simulink model "gm_rec_i2s"  (R2023b)
settings: Solver=VariableStepAuto  StartTime=0.0  StopTime=20  RelTol=1e-3
undefined symbols (not defined in the file or in its folder): cnt1_LRCLK, cnt2_SCLK
libraries: hdlsllib x4
(part 3 of 4)

== system gm_rec_i2s/REC_I2S_NOFIFO/Subsystem1/SIPO_16BIT/SIPO_8BIT/SIPO_4BIT/SIPO_2BIT ==
  SERIAL_IN : Inport  OutDataTypeStr=boolean
  ENABLE : Inport  Port=2
  Bus Creator : BusCreator  Inputs=2
  Delay : Delay  DelayLength=1  InitialCondition=0  ShowEnablePort=on
      settings: InputPortMap=u0,e6
  Delay1 : Delay  DelayLength=1  InitialCondition=0  ShowEnablePort=on
      settings: InputPortMap=u0,e6
  PARA_OUT : Outport  OutDataTypeStr=boolean  VectorParamsAs1DForOutWhenUnconnected=off
  SERIAL_OUT : Outport  Port=2  OutDataTypeStr=boolean  VectorParamsAs1DForOutWhenUnconnected=off
  wires:
  Bus Creator/1 -> PARA_OUT/1
  Delay/1 -> Delay1/1, Bus Creator/2
  Delay1/1 -> Bus Creator/1, SERIAL_OUT/1
  ENABLE/1 -> Delay/2, Delay1/2
  SERIAL_IN/1 -> Delay/1

== system gm_rec_i2s/REC_I2S_NOFIFO/Subsystem1/SIPO_16BIT/SIPO_8BIT/SIPO_4BIT/SIPO_2BIT1 ==
  SERIAL_IN : Inport
  ENABLE : Inport  Port=2
  Bus Creator : BusCreator  Inputs=2
  Delay : Delay  DelayLength=1  InitialCondition=0  ShowEnablePort=on
      settings: InputPortMap=u0,e6
  Delay1 : Delay  DelayLength=1  InitialCondition=0  ShowEnablePort=on
      settings: InputPortMap=u0,e6
  PARA_OUT : Outport  VectorParamsAs1DForOutWhenUnconnected=off
  SERIAL_OUT : Outport  Port=2  VectorParamsAs1DForOutWhenUnconnected=off
  wires:
  Bus Creator/1 -> PARA_OUT/1
  Delay/1 -> Delay1/1, Bus Creator/2
  Delay1/1 -> Bus Creator/1, SERIAL_OUT/1
  ENABLE/1 -> Delay/2, Delay1/2
  SERIAL_IN/1 -> Delay/1

== system gm_rec_i2s/REC_I2S_NOFIFO/Subsystem1/SIPO_16BIT/SIPO_8BIT/SIPO_4BIT1/SIPO_2BIT ==
  SERIAL_IN : Inport
  ENABLE : Inport  Port=2
  Bus Creator : BusCreator  Inputs=2
  Delay : Delay  DelayLength=1  InitialCondition=0  ShowEnablePort=on
      settings: InputPortMap=u0,e6
  Delay1 : Delay  DelayLength=1  InitialCondition=0  ShowEnablePort=on
      settings: InputPortMap=u0,e6
  PARA_OUT : Outport  VectorParamsAs1DForOutWhenUnconnected=off
  SERIAL_OUT : Outport  Port=2  VectorParamsAs1DForOutWhenUnconnected=off
  wires:
  Bus Creator/1 -> PARA_OUT/1
  Delay/1 -> Delay1/1, Bus Creator/2
  Delay1/1 -> Bus Creator/1, SERIAL_OUT/1
  ENABLE/1 -> Delay/2, Delay1/2
  SERIAL_IN/1 -> Delay/1

== system gm_rec_i2s/REC_I2S_NOFIFO/Subsystem1/SIPO_16BIT/SIPO_8BIT/SIPO_4BIT1/SIPO_2BIT1 ==
  SERIAL_IN : Inport
  ENABLE : Inport  Port=2
  Bus Creator : BusCreator  Inputs=2
  Delay : Delay  DelayLength=1  InitialCondition=0  ShowEnablePort=on
      settings: InputPortMap=u0,e6
  Delay1 : Delay  DelayLength=1  InitialCondition=0  ShowEnablePort=on
      settings: InputPortMap=u0,e6
  PARA_OUT : Outport  VectorParamsAs1DForOutWhenUnconnected=off
  SERIAL_OUT : Outport  Port=2  VectorParamsAs1DForOutWhenUnconnected=off
  wires:
  Bus Creator/1 -> PARA_OUT/1
  Delay/1 -> Delay1/1, Bus Creator/2
  Delay1/1 -> Bus Creator/1, SERIAL_OUT/1
  ENABLE/1 -> Delay/2, Delay1/2
  SERIAL_IN/1 -> Delay/1

== system gm_rec_i2s/REC_I2S_NOFIFO/Subsystem1/SIPO_16BIT/SIPO_8BIT1/SIPO_4BIT/SIPO_2BIT ==
  SERIAL_IN : Inport
  ENABLE : Inport  Port=2
  Bus Creator : BusCreator  Inputs=2
  Delay : Delay  DelayLength=1  InitialCondition=0  ShowEnablePort=on
      settings: InputPortMap=u0,e6
  Delay1 : Delay  DelayLength=1  InitialCondition=0  ShowEnablePort=on
      settings: InputPortMap=u0,e6
  PARA_OUT : Outport  VectorParamsAs1DForOutWhenUnconnected=off
  SERIAL_OUT : Outport  Port=2  VectorParamsAs1DForOutWhenUnconnected=off
  wires:
  Bus Creator/1 -> PARA_OUT/1
  Delay/1 -> Delay1/1, Bus Creator/2
  Delay1/1 -> Bus Creator/1, SERIAL_OUT/1
  ENABLE/1 -> Delay/2, Delay1/2
  SERIAL_IN/1 -> Delay/1

== system gm_rec_i2s/REC_I2S_NOFIFO/Subsystem1/SIPO_16BIT/SIPO_8BIT1/SIPO_4BIT/SIPO_2BIT1 ==
  SERIAL_IN : Inport
  ENABLE : Inport  Port=2
  Bus Creator : BusCreator  Inputs=2
  Delay : Delay  DelayLength=1  InitialCondition=0  ShowEnablePort=on
      settings: InputPortMap=u0,e6
  Delay1 : Delay  DelayLength=1  InitialCondition=0  ShowEnablePort=on
      settings: InputPortMap=u0,e6
  PARA_OUT : Outport  VectorParamsAs1DForOutWhenUnconnected=off
  SERIAL_OUT : Outport  Port=2  VectorParamsAs1DForOutWhenUnconnected=off
  wires:
  Bus Creator/1 -> PARA_OUT/1
  Delay/1 -> Delay1/1, Bus Creator/2
  Delay1/1 -> Bus Creator/1, SERIAL_OUT/1
  ENABLE/1 -> Delay/2, Delay1/2
  SERIAL_IN/1 -> Delay/1

== system gm_rec_i2s/REC_I2S_NOFIFO/Subsystem1/SIPO_16BIT/SIPO_8BIT1/SIPO_4BIT1/SIPO_2BIT ==
  SERIAL_IN : Inport
  ENABLE : Inport  Port=2
  Bus Creator : BusCreator  Inputs=2
  Delay : Delay  DelayLength=1  InitialCondition=0  ShowEnablePort=on
      settings: InputPortMap=u0,e6
  Delay1 : Delay  DelayLength=1  InitialCondition=0  ShowEnablePort=on
      settings: InputPortMap=u0,e6
  PARA_OUT : Outport  VectorParamsAs1DForOutWhenUnconnected=off
  SERIAL_OUT : Outport  Port=2  VectorParamsAs1DForOutWhenUnconnected=off
  wires:
  Bus Creator/1 -> PARA_OUT/1
  Delay/1 -> Delay1/1, Bus Creator/2
  Delay1/1 -> Bus Creator/1, SERIAL_OUT/1
  ENABLE/1 -> Delay/2, Delay1/2
  SERIAL_IN/1 -> Delay/1

== system gm_rec_i2s/REC_I2S_NOFIFO/Subsystem1/SIPO_16BIT/SIPO_8BIT1/SIPO_4BIT1/SIPO_2BIT1 ==
  SERIAL_IN : Inport
  ENABLE : Inport  Port=2
  Bus Creator : BusCreator  Inputs=2
  Delay : Delay  DelayLength=1  InitialCondition=0  ShowEnablePort=on
      settings: InputPortMap=u0,e6
  Delay1 : Delay  DelayLength=1  InitialCondition=0  ShowEnablePort=on
      settings: InputPortMap=u0,e6
  PARA_OUT : Outport  VectorParamsAs1DForOutWhenUnconnected=off
  SERIAL_OUT : Outport  Port=2  VectorParamsAs1DForOutWhenUnconnected=off
  wires:
  Bus Creator/1 -> PARA_OUT/1
  Delay/1 -> Delay1/1, Bus Creator/2
  Delay1/1 -> Bus Creator/1, SERIAL_OUT/1
  ENABLE/1 -> Delay/2, Delay1/2
  SERIAL_IN/1 -> Delay/1

== system gm_rec_i2s/REC_I2S_NOFIFO/Subsystem1/SIPO_16BIT1/SIPO_8BIT/SIPO_4BIT/SIPO_2BIT ==
  SERIAL_IN : Inport  OutDataTypeStr=boolean
  ENABLE : Inport  Port=2
  Bus Creator : BusCreator  Inputs=2
  Delay : Delay  DelayLength=1  InitialCondition=0  ShowEnablePort=on
      settings: InputPortMap=u0,e6
  Delay1 : Delay  DelayLength=1  InitialCondition=0  ShowEnablePort=on
      settings: InputPortMap=u0,e6
  PARA_OUT : Outport  OutDataTypeStr=boolean  VectorParamsAs1DForOutWhenUnconnected=off
  SERIAL_OUT : Outport  Port=2  OutDataTypeStr=boolean  VectorParamsAs1DForOutWhenUnconnected=off
  wires:
  Bus Creator/1 -> PARA_OUT/1
  Delay/1 -> Delay1/1, Bus Creator/2
  Delay1/1 -> Bus Creator/1, SERIAL_OUT/1
  ENABLE/1 -> Delay/2, Delay1/2
  SERIAL_IN/1 -> Delay/1

== system gm_rec_i2s/REC_I2S_NOFIFO/Subsystem1/SIPO_16BIT1/SIPO_8BIT/SIPO_4BIT/SIPO_2BIT1 ==
  SERIAL_IN : Inport
  ENABLE : Inport  Port=2
  Bus Creator : BusCreator  Inputs=2
  Delay : Delay  DelayLength=1  InitialCondition=0  ShowEnablePort=on
      settings: InputPortMap=u0,e6
  Delay1 : Delay  DelayLength=1  InitialCondition=0  ShowEnablePort=on
      settings: InputPortMap=u0,e6
  PARA_OUT : Outport  VectorParamsAs1DForOutWhenUnconnected=off
  SERIAL_OUT : Outport  Port=2  VectorParamsAs1DForOutWhenUnconnected=off
  wires:
  Bus Creator/1 -> PARA_OUT/1
  Delay/1 -> Delay1/1, Bus Creator/2
  Delay1/1 -> Bus Creator/1, SERIAL_OUT/1
  ENABLE/1 -> Delay/2, Delay1/2
  SERIAL_IN/1 -> Delay/1

== system gm_rec_i2s/REC_I2S_NOFIFO/Subsystem1/SIPO_16BIT1/SIPO_8BIT/SIPO_4BIT1/SIPO_2BIT ==
  SERIAL_IN : Inport
  ENABLE : Inport  Port=2
  Bus Creator : BusCreator  Inputs=2
  Delay : Delay  DelayLength=1  InitialCondition=0  ShowEnablePort=on
      settings: InputPortMap=u0,e6
  Delay1 : Delay  DelayLength=1  InitialCondition=0  ShowEnablePort=on
      settings: InputPortMap=u0,e6
  PARA_OUT : Outport  VectorParamsAs1DForOutWhenUnconnected=off
  SERIAL_OUT : Outport  Port=2  VectorParamsAs1DForOutWhenUnconnected=off
  wires:
  Bus Creator/1 -> PARA_OUT/1
  Delay/1 -> Delay1/1, Bus Creator/2
  Delay1/1 -> Bus Creator/1, SERIAL_OUT/1
  ENABLE/1 -> Delay/2, Delay1/2
  SERIAL_IN/1 -> Delay/1

== system gm_rec_i2s/REC_I2S_NOFIFO/Subsystem1/SIPO_16BIT1/SIPO_8BIT/SIPO_4BIT1/SIPO_2BIT1 ==
  SERIAL_IN : Inport
  ENABLE : Inport  Port=2
  Bus Creator : BusCreator  Inputs=2
  Delay : Delay  DelayLength=1  InitialCondition=0  ShowEnablePort=on
      settings: InputPortMap=u0,e6
  Delay1 : Delay  DelayLength=1  InitialCondition=0  ShowEnablePort=on
      settings: InputPortMap=u0,e6
  PARA_OUT : Outport  VectorParamsAs1DForOutWhenUnconnected=off
  SERIAL_OUT : Outport  Port=2  VectorParamsAs1DForOutWhenUnconnected=off
  wires:
  Bus Creator/1 -> PARA_OUT/1
  Delay/1 -> Delay1/1, Bus Creator/2
  Delay1/1 -> Bus Creator/1, SERIAL_OUT/1
  ENABLE/1 -> Delay/2, Delay1/2
  SERIAL_IN/1 -> Delay/1

== system gm_rec_i2s/REC_I2S_NOFIFO/Subsystem1/SIPO_16BIT1/SIPO_8BIT1/SIPO_4BIT/SIPO_2BIT ==
  SERIAL_IN : Inport
  ENABLE : Inport  Port=2
  Bus Creator : BusCreator  Inputs=2
  Delay : Delay  DelayLength=1  InitialCondition=0  ShowEnablePort=on
      settings: InputPortMap=u0,e6
  Delay1 : Delay  DelayLength=1  InitialCondition=0  ShowEnablePort=on
      settings: InputPortMap=u0,e6
  PARA_OUT : Outport  VectorParamsAs1DForOutWhenUnconnected=off
  SERIAL_OUT : Outport  Port=2  VectorParamsAs1DForOutWhenUnconnected=off
  wires:
  Bus Creator/1 -> PARA_OUT/1
  Delay/1 -> Delay1/1, Bus Creator/2
  Delay1/1 -> Bus Creator/1, SERIAL_OUT/1
  ENABLE/1 -> Delay/2, Delay1/2
  SERIAL_IN/1 -> Delay/1

== system gm_rec_i2s/REC_I2S_NOFIFO/Subsystem1/SIPO_16BIT1/SIPO_8BIT1/SIPO_4BIT/SIPO_2BIT1 ==
  SERIAL_IN : Inport
  ENABLE : Inport  Port=2
  Bus Creator : BusCreator  Inputs=2
  Delay : Delay  DelayLength=1  InitialCondition=0  ShowEnablePort=on
      settings: InputPortMap=u0,e6
  Delay1 : Delay  DelayLength=1  InitialCondition=0  ShowEnablePort=on
      settings: InputPortMap=u0,e6
  PARA_OUT : Outport  VectorParamsAs1DForOutWhenUnconnected=off
  SERIAL_OUT : Outport  Port=2  VectorParamsAs1DForOutWhenUnconnected=off
  wires:
  Bus Creator/1 -> PARA_OUT/1
  Delay/1 -> Delay1/1, Bus Creator/2
  Delay1/1 -> Bus Creator/1, SERIAL_OUT/1
  ENABLE/1 -> Delay/2, Delay1/2
  SERIAL_IN/1 -> Delay/1

== system gm_rec_i2s/REC_I2S_NOFIFO/Subsystem1/SIPO_16BIT1/SIPO_8BIT1/SIPO_4BIT1/SIPO_2BIT ==
  SERIAL_IN : Inport
  ENABLE : Inport  Port=2
  Bus Creator : BusCreator  Inputs=2
  Delay : Delay  DelayLength=1  InitialCondition=0  ShowEnablePort=on
      settings: InputPortMap=u0,e6
  Delay1 : Delay  DelayLength=1  InitialCondition=0  ShowEnablePort=on
      settings: InputPortMap=u0,e6
  PARA_OUT : Outport  VectorParamsAs1DForOutWhenUnconnected=off
  SERIAL_OUT : Outport  Port=2  VectorParamsAs1DForOutWhenUnconnected=off
  wires:
  Bus Creator/1 -> PARA_OUT/1
  Delay/1 -> Delay1/1, Bus Creator/2
  Delay1/1 -> Bus Creator/1, SERIAL_OUT/1
  ENABLE/1 -> Delay/2, Delay1/2
  SERIAL_IN/1 -> Delay/1

== system gm_rec_i2s/REC_I2S_NOFIFO/Subsystem1/SIPO_16BIT1/SIPO_8BIT1/SIPO_4BIT1/SIPO_2BIT1 ==
  SERIAL_IN : Inport
  ENABLE : Inport  Port=2
  Bus Creator : BusCreator  Inputs=2
  Delay : Delay  DelayLength=1  InitialCondition=0  ShowEnablePort=on
      settings: InputPortMap=u0,e6
  Delay1 : Delay  DelayLength=1  InitialCondition=0  ShowEnablePort=on
      settings: InputPortMap=u0,e6
  PARA_OUT : Outport  VectorParamsAs1DForOutWhenUnconnected=off
  SERIAL_OUT : Outport  Port=2  VectorParamsAs1DForOutWhenUnconnected=off
  wires:
  Bus Creator/1 -> PARA_OUT/1
  Delay/1 -> Delay1/1, Bus Creator/2
  Delay1/1 -> Bus Creator/1, SERIAL_OUT/1
  ENABLE/1 -> Delay/2, Delay1/2
  SERIAL_IN/1 -> Delay/1

== system gm_rec_i2s/REC_I2S_FIFO/SIPO_32BIT_L/Subsystem/SIPO_16BIT/SIPO_8BIT/SIPO_4BIT/2BIT_SIPO ==
  SERIAL_IN : Inport
  Constant : Constant  OutDataTypeStr=boolean  SampleTime=-1
  Delay : Delay  DelayLength=1  InitialCondition=0  ShowEnablePort=on
      settings: InputPortMap=u0,e6
  Delay1 : Delay  DelayLength=1  InitialCondition=0  ShowEnablePort=on
      settings: InputPortMap=u0,e6
  Vector Concatenate : Concatenate
  PARA_OUT : Outport  VectorParamsAs1DForOutWhenUnconnected=off
  SERIAL_OUT : Outport  Port=2  VectorParamsAs1DForOutWhenUnconnected=off
  wires:
  SERIAL_IN/1 -> Delay/1
  Delay1/1 -> SERIAL_OUT/1, Vector Concatenate/1
  Vector Concatenate/1 -> PARA_OUT/1
  Delay/1 -> Vector Concatenate/2, Delay1/1
  Constant/1 -> Delay1/2, Delay/2

== system gm_rec_i2s/REC_I2S_FIFO/SIPO_32BIT_L/Subsystem/SIPO_16BIT/SIPO_8BIT/SIPO_4BIT/2BIT_SIPO1 ==
  SERIAL_IN : Inport
  Constant : Constant  OutDataTypeStr=boolean  SampleTime=-1
  Delay : Delay  DelayLength=1  InitialCondition=0  ShowEnablePort=on
      settings: InputPortMap=u0,e6
  Delay1 : Delay  DelayLength=1  InitialCondition=0  ShowEnablePort=on
      settings: InputPortMap=u0,e6
  Vector Concatenate : Concatenate
  PARA_OUT : Outport  VectorParamsAs1DForOutWhenUnconnected=off
  SERIAL_OUT : Outport  Port=2  VectorParamsAs1DForOutWhenUnconnected=off
  wires:
  SERIAL_IN/1 -> Delay/1
  Delay1/1 -> SERIAL_OUT/1, Vector Concatenate/1
  Vector Concatenate/1 -> PARA_OUT/1
  Delay/1 -> Vector Concatenate/2, Delay1/1
  Constant/1 -> Delay1/2, Delay/2

== system gm_rec_i2s/REC_I2S_FIFO/SIPO_32BIT_L/Subsystem/SIPO_16BIT/SIPO_8BIT/SIPO_4BIT1/2BIT_SIPO ==
  SERIAL_IN : Inport
  Constant : Constant  OutDataTypeStr=boolean  SampleTime=-1
  Delay : Delay  DelayLength=1  InitialCondition=0  ShowEnablePort=on
      settings: InputPortMap=u0,e6
  Delay1 : Delay  DelayLength=1  InitialCondition=0  ShowEnablePort=on
      settings: InputPortMap=u0,e6
  Vector Concatenate : Concatenate
  PARA_OUT : Outport  VectorParamsAs1DForOutWhenUnconnected=off
  SERIAL_OUT : Outport  Port=2  VectorParamsAs1DForOutWhenUnconnected=off
  wires:
  SERIAL_IN/1 -> Delay/1
  Delay1/1 -> SERIAL_OUT/1, Vector Concatenate/1
  Vector Concatenate/1 -> PARA_OUT/1
  Delay/1 -> Vector Concatenate/2, Delay1/1
  Constant/1 -> Delay1/2, Delay/2

== system gm_rec_i2s/REC_I2S_FIFO/SIPO_32BIT_L/Subsystem/SIPO_16BIT/SIPO_8BIT/SIPO_4BIT1/2BIT_SIPO1 ==
  SERIAL_IN : Inport
  Constant : Constant  OutDataTypeStr=boolean  SampleTime=-1
  Delay : Delay  DelayLength=1  InitialCondition=0  ShowEnablePort=on
      settings: InputPortMap=u0,e6
  Delay1 : Delay  DelayLength=1  InitialCondition=0  ShowEnablePort=on
      settings: InputPortMap=u0,e6
  Vector Concatenate : Concatenate
  PARA_OUT : Outport  VectorParamsAs1DForOutWhenUnconnected=off
  SERIAL_OUT : Outport  Port=2  VectorParamsAs1DForOutWhenUnconnected=off
  wires:
  SERIAL_IN/1 -> Delay/1
  Delay1/1 -> SERIAL_OUT/1, Vector Concatenate/1
  Vector Concatenate/1 -> PARA_OUT/1
  Delay/1 -> Vector Concatenate/2, Delay1/1
  Constant/1 -> Delay1/2, Delay/2

== system gm_rec_i2s/REC_I2S_FIFO/SIPO_32BIT_L/Subsystem/SIPO_16BIT/SIPO_8BIT1/SIPO_4BIT/2BIT_SIPO ==
  SERIAL_IN : Inport
  Constant : Constant  OutDataTypeStr=boolean  SampleTime=-1
  Delay : Delay  DelayLength=1  InitialCondition=0  ShowEnablePort=on
      settings: InputPortMap=u0,e6
  Delay1 : Delay  DelayLength=1  InitialCondition=0  ShowEnablePort=on
      settings: InputPortMap=u0,e6
  Vector Concatenate : Concatenate
  PARA_OUT : Outport  VectorParamsAs1DForOutWhenUnconnected=off
  SERIAL_OUT : Outport  Port=2  VectorParamsAs1DForOutWhenUnconnected=off
  wires:
  SERIAL_IN/1 -> Delay/1
  Delay1/1 -> SERIAL_OUT/1, Vector Concatenate/1
  Vector Concatenate/1 -> PARA_OUT/1
  Delay/1 -> Vector Concatenate/2, Delay1/1
  Constant/1 -> Delay1/2, Delay/2

== system gm_rec_i2s/REC_I2S_FIFO/SIPO_32BIT_L/Subsystem/SIPO_16BIT/SIPO_8BIT1/SIPO_4BIT/2BIT_SIPO1 ==
  SERIAL_IN : Inport
  Constant : Constant  OutDataTypeStr=boolean  SampleTime=-1
  Delay : Delay  DelayLength=1  InitialCondition=0  ShowEnablePort=on
      settings: InputPortMap=u0,e6
  Delay1 : Delay  DelayLength=1  InitialCondition=0  ShowEnablePort=on
      settings: InputPortMap=u0,e6
  Vector Concatenate : Concatenate
  PARA_OUT : Outport  VectorParamsAs1DForOutWhenUnconnected=off
  SERIAL_OUT : Outport  Port=2  VectorParamsAs1DForOutWhenUnconnected=off
  wires:
  SERIAL_IN/1 -> Delay/1
  Delay1/1 -> SERIAL_OUT/1, Vector Concatenate/1
  Vector Concatenate/1 -> PARA_OUT/1
  Delay/1 -> Vector Concatenate/2, Delay1/1
  Constant/1 -> Delay1/2, Delay/2

== system gm_rec_i2s/REC_I2S_FIFO/SIPO_32BIT_L/Subsystem/SIPO_16BIT/SIPO_8BIT1/SIPO_4BIT1/2BIT_SIPO ==
  SERIAL_IN : Inport
  Constant : Constant  OutDataTypeStr=boolean  SampleTime=-1
  Delay : Delay  DelayLength=1  InitialCondition=0  ShowEnablePort=on
      settings: InputPortMap=u0,e6
  Delay1 : Delay  DelayLength=1  InitialCondition=0  ShowEnablePort=on
      settings: InputPortMap=u0,e6
  Vector Concatenate : Concatenate
  PARA_OUT : Outport  VectorParamsAs1DForOutWhenUnconnected=off
  SERIAL_OUT : Outport  Port=2  VectorParamsAs1DForOutWhenUnconnected=off
  wires:
  SERIAL_IN/1 -> Delay/1
  Delay1/1 -> SERIAL_OUT/1, Vector Concatenate/1
  Vector Concatenate/1 -> PARA_OUT/1
  Delay/1 -> Vector Concatenate/2, Delay1/1
  Constant/1 -> Delay1/2, Delay/2

== system gm_rec_i2s/REC_I2S_FIFO/SIPO_32BIT_L/Subsystem/SIPO_16BIT/SIPO_8BIT1/SIPO_4BIT1/2BIT_SIPO1 ==
  SERIAL_IN : Inport
  Constant : Constant  OutDataTypeStr=boolean  SampleTime=-1
  Delay : Delay  DelayLength=1  InitialCondition=0  ShowEnablePort=on
      settings: InputPortMap=u0,e6
  Delay1 : Delay  DelayLength=1  InitialCondition=0  ShowEnablePort=on
      settings: InputPortMap=u0,e6
  Vector Concatenate : Concatenate
  PARA_OUT : Outport  VectorParamsAs1DForOutWhenUnconnected=off
  SERIAL_OUT : Outport  Port=2  VectorParamsAs1DForOutWhenUnconnected=off
  wires:
  SERIAL_IN/1 -> Delay/1
  Delay1/1 -> SERIAL_OUT/1, Vector Concatenate/1
  Vector Concatenate/1 -> PARA_OUT/1
  Delay/1 -> Vector Concatenate/2, Delay1/1
  Constant/1 -> Delay1/2, Delay/2

== system gm_rec_i2s/REC_I2S_FIFO/SIPO_32BIT_L/Subsystem/SIPO_16BIT1/SIPO_8BIT/SIPO_4BIT/2BIT_SIPO ==
  SERIAL_IN : Inport
  Constant : Constant  OutDataTypeStr=boolean  SampleTime=-1
  Delay : Delay  DelayLength=1  InitialCondition=0  ShowEnablePort=on
      settings: InputPortMap=u0,e6
  Delay1 : Delay  DelayLength=1  InitialCondition=0  ShowEnablePort=on
      settings: InputPortMap=u0,e6
  Vector Concatenate : Concatenate
  PARA_OUT : Outport  VectorParamsAs1DForOutWhenUnconnected=off
  SERIAL_OUT : Outport  Port=2  VectorParamsAs1DForOutWhenUnconnected=off
  wires:
  SERIAL_IN/1 -> Delay/1
  Delay1/1 -> SERIAL_OUT/1, Vector Concatenate/1
  Vector Concatenate/1 -> PARA_OUT/1
  Delay/1 -> Vector Concatenate/2, Delay1/1
  Constant/1 -> Delay1/2, Delay/2

== system gm_rec_i2s/REC_I2S_FIFO/SIPO_32BIT_L/Subsystem/SIPO_16BIT1/SIPO_8BIT/SIPO_4BIT/2BIT_SIPO1 ==
  SERIAL_IN : Inport
  Constant : Constant  OutDataTypeStr=boolean  SampleTime=-1
  Delay : Delay  DelayLength=1  InitialCondition=0  ShowEnablePort=on
      settings: InputPortMap=u0,e6
  Delay1 : Delay  DelayLength=1  InitialCondition=0  ShowEnablePort=on
      settings: InputPortMap=u0,e6
  Vector Concatenate : Concatenate
  PARA_OUT : Outport  VectorParamsAs1DForOutWhenUnconnected=off
  SERIAL_OUT : Outport  Port=2  VectorParamsAs1DForOutWhenUnconnected=off
  wires:
  SERIAL_IN/1 -> Delay/1
  Delay1/1 -> SERIAL_OUT/1, Vector Concatenate/1
  Vector Concatenate/1 -> PARA_OUT/1
  Delay/1 -> Vector Concatenate/2, Delay1/1
  Constant/1 -> Delay1/2, Delay/2

== system gm_rec_i2s/REC_I2S_FIFO/SIPO_32BIT_L/Subsystem/SIPO_16BIT1/SIPO_8BIT/SIPO_4BIT1/2BIT_SIPO ==
  SERIAL_IN : Inport
  Constant : Constant  OutDataTypeStr=boolean  SampleTime=-1
  Delay : Delay  DelayLength=1  InitialCondition=0  ShowEnablePort=on
      settings: InputPortMap=u0,e6
  Delay1 : Delay  DelayLength=1  InitialCondition=0  ShowEnablePort=on
      settings: InputPortMap=u0,e6
  Vector Concatenate : Concatenate
  PARA_OUT : Outport  VectorParamsAs1DForOutWhenUnconnected=off
  SERIAL_OUT : Outport  Port=2  VectorParamsAs1DForOutWhenUnconnected=off
  wires:
  SERIAL_IN/1 -> Delay/1
  Delay1/1 -> SERIAL_OUT/1, Vector Concatenate/1
  Vector Concatenate/1 -> PARA_OUT/1
  Delay/1 -> Vector Concatenate/2, Delay1/1
  Constant/1 -> Delay1/2, Delay/2

== system gm_rec_i2s/REC_I2S_FIFO/SIPO_32BIT_L/Subsystem/SIPO_16BIT1/SIPO_8BIT/SIPO_4BIT1/2BIT_SIPO1 ==
  SERIAL_IN : Inport
  Constant : Constant  OutDataTypeStr=boolean  SampleTime=-1
  Delay : Delay  DelayLength=1  InitialCondition=0  ShowEnablePort=on
      settings: InputPortMap=u0,e6
  Delay1 : Delay  DelayLength=1  InitialCondition=0  ShowEnablePort=on
      settings: InputPortMap=u0,e6
  Vector Concatenate : Concatenate
  PARA_OUT : Outport  VectorParamsAs1DForOutWhenUnconnected=off
  SERIAL_OUT : Outport  Port=2  VectorParamsAs1DForOutWhenUnconnected=off
  wires:
  SERIAL_IN/1 -> Delay/1
  Delay1/1 -> SERIAL_OUT/1, Vector Concatenate/1
  Vector Concatenate/1 -> PARA_OUT/1
  Delay/1 -> Vector Concatenate/2, Delay1/1
  Constant/1 -> Delay1/2, Delay/2

== system gm_rec_i2s/REC_I2S_FIFO/SIPO_32BIT_L/Subsystem/SIPO_16BIT1/SIPO_8BIT1/SIPO_4BIT/2BIT_SIPO ==
  SERIAL_IN : Inport
  Constant : Constant  OutDataTypeStr=boolean  SampleTime=-1
  Delay : Delay  DelayLength=1  InitialCondition=0  ShowEnablePort=on
      settings: InputPortMap=u0,e6
  Delay1 : Delay  DelayLength=1  InitialCondition=0  ShowEnablePort=on
      settings: InputPortMap=u0,e6
  Vector Concatenate : Concatenate
  PARA_OUT : Outport  VectorParamsAs1DForOutWhenUnconnected=off
  SERIAL_OUT : Outport  Port=2  VectorParamsAs1DForOutWhenUnconnected=off
  wires:
  SERIAL_IN/1 -> Delay/1
  Delay1/1 -> SERIAL_OUT/1, Vector Concatenate/1
  Vector Concatenate/1 -> PARA_OUT/1
  Delay/1 -> Vector Concatenate/2, Delay1/1
  Constant/1 -> Delay1/2, Delay/2

== system gm_rec_i2s/REC_I2S_FIFO/SIPO_32BIT_L/Subsystem/SIPO_16BIT1/SIPO_8BIT1/SIPO_4BIT/2BIT_SIPO1 ==
  SERIAL_IN : Inport
  Constant : Constant  OutDataTypeStr=boolean  SampleTime=-1
  Delay : Delay  DelayLength=1  InitialCondition=0  ShowEnablePort=on
      settings: InputPortMap=u0,e6
  Delay1 : Delay  DelayLength=1  InitialCondition=0  ShowEnablePort=on
      settings: InputPortMap=u0,e6
  Vector Concatenate : Concatenate
  PARA_OUT : Outport  VectorParamsAs1DForOutWhenUnconnected=off
  SERIAL_OUT : Outport  Port=2  VectorParamsAs1DForOutWhenUnconnected=off
  wires:
  SERIAL_IN/1 -> Delay/1
  Delay1/1 -> SERIAL_OUT/1, Vector Concatenate/1
  Vector Concatenate/1 -> PARA_OUT/1
  Delay/1 -> Vector Concatenate/2, Delay1/1
  Constant/1 -> Delay1/2, Delay/2

== system gm_rec_i2s/REC_I2S_FIFO/SIPO_32BIT_L/Subsystem/SIPO_16BIT1/SIPO_8BIT1/SIPO_4BIT1/2BIT_SIPO ==
  SERIAL_IN : Inport
  Constant : Constant  OutDataTypeStr=boolean  SampleTime=-1
  Delay : Delay  DelayLength=1  InitialCondition=0  ShowEnablePort=on
      settings: InputPortMap=u0,e6
  Delay1 : Delay  DelayLength=1  InitialCondition=0  ShowEnablePort=on
      settings: InputPortMap=u0,e6
  Vector Concatenate : Concatenate
  PARA_OUT : Outport  VectorParamsAs1DForOutWhenUnconnected=off
  SERIAL_OUT : Outport  Port=2  VectorParamsAs1DForOutWhenUnconnected=off
  wires:
  SERIAL_IN/1 -> Delay/1
  Delay1/1 -> SERIAL_OUT/1, Vector Concatenate/1
  Vector Concatenate/1 -> PARA_OUT/1
  Delay/1 -> Vector Concatenate/2, Delay1/1
  Constant/1 -> Delay1/2, Delay/2

== system gm_rec_i2s/REC_I2S_FIFO/SIPO_32BIT_L/Subsystem/SIPO_16BIT1/SIPO_8BIT1/SIPO_4BIT1/2BIT_SIPO1 ==
  SERIAL_IN : Inport
  Constant : Constant  OutDataTypeStr=boolean  SampleTime=-1
  Delay : Delay  DelayLength=1  InitialCondition=0  ShowEnablePort=on
      settings: InputPortMap=u0,e6
  Delay1 : Delay  DelayLength=1  InitialCondition=0  ShowEnablePort=on
      settings: InputPortMap=u0,e6
  Vector Concatenate : Concatenate
  PARA_OUT : Outport  VectorParamsAs1DForOutWhenUnconnected=off
  SERIAL_OUT : Outport  Port=2  VectorParamsAs1DForOutWhenUnconnected=off
  wires:
  SERIAL_IN/1 -> Delay/1
  Delay1/1 -> SERIAL_OUT/1, Vector Concatenate/1
  Vector Concatenate/1 -> PARA_OUT/1
  Delay/1 -> Vector Concatenate/2, Delay1/1
  Constant/1 -> Delay1/2, Delay/2

== system gm_rec_i2s/REC_I2S_FIFO/SIPO_32BIT_R/Subsystem/SIPO_16BIT/SIPO_8BIT/SIPO_4BIT/2BIT_SIPO ==
  SERIAL_IN : Inport
  Constant : Constant  OutDataTypeStr=boolean  SampleTime=-1
  Delay : Delay  DelayLength=1  InitialCondition=0  ShowEnablePort=on
      settings: InputPortMap=u0,e6
  Delay1 : Delay  DelayLength=1  InitialCondition=0  ShowEnablePort=on
      settings: InputPortMap=u0,e6
  Vector Concatenate : Concatenate
  PARA_OUT : Outport  VectorParamsAs1DForOutWhenUnconnected=off
  SERIAL_OUT : Outport  Port=2  VectorParamsAs1DForOutWhenUnconnected=off
  wires:
  SERIAL_IN/1 -> Delay/1
  Delay1/1 -> SERIAL_OUT/1, Vector Concatenate/1
  Vector Concatenate/1 -> PARA_OUT/1
  Delay/1 -> Vector Concatenate/2, Delay1/1
  Constant/1 -> Delay1/2, Delay/2

== system gm_rec_i2s/REC_I2S_FIFO/SIPO_32BIT_R/Subsystem/SIPO_16BIT/SIPO_8BIT/SIPO_4BIT/2BIT_SIPO1 ==
  SERIAL_IN : Inport
  Constant : Constant  OutDataTypeStr=boolean  SampleTime=-1
  Delay : Delay  DelayLength=1  InitialCondition=0  ShowEnablePort=on
      settings: InputPortMap=u0,e6
  Delay1 : Delay  DelayLength=1  InitialCondition=0  ShowEnablePort=on
      settings: InputPortMap=u0,e6
  Vector Concatenate : Concatenate
  PARA_OUT : Outport  VectorParamsAs1DForOutWhenUnconnected=off
  SERIAL_OUT : Outport  Port=2  VectorParamsAs1DForOutWhenUnconnected=off
  wires:
  SERIAL_IN/1 -> Delay/1
  Delay1/1 -> SERIAL_OUT/1, Vector Concatenate/1
  Vector Concatenate/1 -> PARA_OUT/1
  Delay/1 -> Vector Concatenate/2, Delay1/1
  Constant/1 -> Delay1/2, Delay/2

== system gm_rec_i2s/REC_I2S_FIFO/SIPO_32BIT_R/Subsystem/SIPO_16BIT/SIPO_8BIT/SIPO_4BIT1/2BIT_SIPO ==
  SERIAL_IN : Inport
  Constant : Constant  OutDataTypeStr=boolean  SampleTime=-1
  Delay : Delay  DelayLength=1  InitialCondition=0  ShowEnablePort=on
      settings: InputPortMap=u0,e6
  Delay1 : Delay  DelayLength=1  InitialCondition=0  ShowEnablePort=on
      settings: InputPortMap=u0,e6
  Vector Concatenate : Concatenate
  PARA_OUT : Outport  VectorParamsAs1DForOutWhenUnconnected=off
  SERIAL_OUT : Outport  Port=2  VectorParamsAs1DForOutWhenUnconnected=off
  wires:
  SERIAL_IN/1 -> Delay/1
  Delay1/1 -> SERIAL_OUT/1, Vector Concatenate/1
  Vector Concatenate/1 -> PARA_OUT/1
  Delay/1 -> Vector Concatenate/2, Delay1/1
  Constant/1 -> Delay1/2, Delay/2

== system gm_rec_i2s/REC_I2S_FIFO/SIPO_32BIT_R/Subsystem/SIPO_16BIT/SIPO_8BIT/SIPO_4BIT1/2BIT_SIPO1 ==
  SERIAL_IN : Inport
  Constant : Constant  OutDataTypeStr=boolean  SampleTime=-1
  Delay : Delay  DelayLength=1  InitialCondition=0  ShowEnablePort=on
      settings: InputPortMap=u0,e6
  Delay1 : Delay  DelayLength=1  InitialCondition=0  ShowEnablePort=on
      settings: InputPortMap=u0,e6
  Vector Concatenate : Concatenate
  PARA_OUT : Outport  VectorParamsAs1DForOutWhenUnconnected=off
  SERIAL_OUT : Outport  Port=2  VectorParamsAs1DForOutWhenUnconnected=off
  wires:
  SERIAL_IN/1 -> Delay/1
  Delay1/1 -> SERIAL_OUT/1, Vector Concatenate/1
  Vector Concatenate/1 -> PARA_OUT/1
  Delay/1 -> Vector Concatenate/2, Delay1/1
  Constant/1 -> Delay1/2, Delay/2

== system gm_rec_i2s/REC_I2S_FIFO/SIPO_32BIT_R/Subsystem/SIPO_16BIT/SIPO_8BIT1/SIPO_4BIT/2BIT_SIPO ==
  SERIAL_IN : Inport
  Constant : Constant  OutDataTypeStr=boolean  SampleTime=-1
  Delay : Delay  DelayLength=1  InitialCondition=0  ShowEnablePort=on
      settings: InputPortMap=u0,e6
  Delay1 : Delay  DelayLength=1  InitialCondition=0  ShowEnablePort=on
      settings: InputPortMap=u0,e6
  Vector Concatenate : Concatenate
  PARA_OUT : Outport  VectorParamsAs1DForOutWhenUnconnected=off
  SERIAL_OUT : Outport  Port=2  VectorParamsAs1DForOutWhenUnconnected=off
  wires:
  SERIAL_IN/1 -> Delay/1
  Delay1/1 -> SERIAL_OUT/1, Vector Concatenate/1
  Vector Concatenate/1 -> PARA_OUT/1
  Delay/1 -> Vector Concatenate/2, Delay1/1
  Constant/1 -> Delay1/2, Delay/2

== system gm_rec_i2s/REC_I2S_FIFO/SIPO_32BIT_R/Subsystem/SIPO_16BIT/SIPO_8BIT1/SIPO_4BIT/2BIT_SIPO1 ==
  SERIAL_IN : Inport
  Constant : Constant  OutDataTypeStr=boolean  SampleTime=-1
  Delay : Delay  DelayLength=1  InitialCondition=0  ShowEnablePort=on
      settings: InputPortMap=u0,e6
  Delay1 : Delay  DelayLength=1  InitialCondition=0  ShowEnablePort=on
      settings: InputPortMap=u0,e6
  Vector Concatenate : Concatenate
  PARA_OUT : Outport  VectorParamsAs1DForOutWhenUnconnected=off
  SERIAL_OUT : Outport  Port=2  VectorParamsAs1DForOutWhenUnconnected=off
  wires:
  SERIAL_IN/1 -> Delay/1
  Delay1/1 -> SERIAL_OUT/1, Vector Concatenate/1
  Vector Concatenate/1 -> PARA_OUT/1
  Delay/1 -> Vector Concatenate/2, Delay1/1
  Constant/1 -> Delay1/2, Delay/2

== system gm_rec_i2s/REC_I2S_FIFO/SIPO_32BIT_R/Subsystem/SIPO_16BIT/SIPO_8BIT1/SIPO_4BIT1/2BIT_SIPO ==
  SERIAL_IN : Inport
  Constant : Constant  OutDataTypeStr=boolean  SampleTime=-1
  Delay : Delay  DelayLength=1  InitialCondition=0  ShowEnablePort=on
      settings: InputPortMap=u0,e6
  Delay1 : Delay  DelayLength=1  InitialCondition=0  ShowEnablePort=on
      settings: InputPortMap=u0,e6
  Vector Concatenate : Concatenate
  PARA_OUT : Outport  VectorParamsAs1DForOutWhenUnconnected=off
  SERIAL_OUT : Outport  Port=2  VectorParamsAs1DForOutWhenUnconnected=off
  wires:
  SERIAL_IN/1 -> Delay/1
  Delay1/1 -> SERIAL_OUT/1, Vector Concatenate/1
  Vector Concatenate/1 -> PARA_OUT/1
  Delay/1 -> Vector Concatenate/2, Delay1/1
  Constant/1 -> Delay1/2, Delay/2

== system gm_rec_i2s/REC_I2S_FIFO/SIPO_32BIT_R/Subsystem/SIPO_16BIT/SIPO_8BIT1/SIPO_4BIT1/2BIT_SIPO1 ==
  SERIAL_IN : Inport
  Constant : Constant  OutDataTypeStr=boolean  SampleTime=-1
  Delay : Delay  DelayLength=1  InitialCondition=0  ShowEnablePort=on
      settings: InputPortMap=u0,e6
  Delay1 : Delay  DelayLength=1  InitialCondition=0  ShowEnablePort=on
      settings: InputPortMap=u0,e6
  Vector Concatenate : Concatenate
  PARA_OUT : Outport  VectorParamsAs1DForOutWhenUnconnected=off
  SERIAL_OUT : Outport  Port=2  VectorParamsAs1DForOutWhenUnconnected=off
  wires:
  SERIAL_IN/1 -> Delay/1
  Delay1/1 -> SERIAL_OUT/1, Vector Concatenate/1
  Vector Concatenate/1 -> PARA_OUT/1
  Delay/1 -> Vector Concatenate/2, Delay1/1
  Constant/1 -> Delay1/2, Delay/2

== system gm_rec_i2s/REC_I2S_FIFO/SIPO_32BIT_R/Subsystem/SIPO_16BIT1/SIPO_8BIT/SIPO_4BIT/2BIT_SIPO ==
  SERIAL_IN : Inport
  Constant : Constant  OutDataTypeStr=boolean  SampleTime=-1
  Delay : Delay  DelayLength=1  InitialCondition=0  ShowEnablePort=on
      settings: InputPortMap=u0,e6
  Delay1 : Delay  DelayLength=1  InitialCondition=0  ShowEnablePort=on
      settings: InputPortMap=u0,e6
  Vector Concatenate : Concatenate
  PARA_OUT : Outport  VectorParamsAs1DForOutWhenUnconnected=off
  SERIAL_OUT : Outport  Port=2  VectorParamsAs1DForOutWhenUnconnected=off
  wires:
  SERIAL_IN/1 -> Delay/1
  Delay1/1 -> SERIAL_OUT/1, Vector Concatenate/1
  Vector Concatenate/1 -> PARA_OUT/1
  Delay/1 -> Vector Concatenate/2, Delay1/1
  Constant/1 -> Delay1/2, Delay/2

== system gm_rec_i2s/REC_I2S_FIFO/SIPO_32BIT_R/Subsystem/SIPO_16BIT1/SIPO_8BIT/SIPO_4BIT/2BIT_SIPO1 ==
  SERIAL_IN : Inport
  Constant : Constant  OutDataTypeStr=boolean  SampleTime=-1
  Delay : Delay  DelayLength=1  InitialCondition=0  ShowEnablePort=on
      settings: InputPortMap=u0,e6
  Delay1 : Delay  DelayLength=1  InitialCondition=0  ShowEnablePort=on
      settings: InputPortMap=u0,e6
  Vector Concatenate : Concatenate
  PARA_OUT : Outport  VectorParamsAs1DForOutWhenUnconnected=off
  SERIAL_OUT : Outport  Port=2  VectorParamsAs1DForOutWhenUnconnected=off
  wires:
  SERIAL_IN/1 -> Delay/1
  Delay1/1 -> SERIAL_OUT/1, Vector Concatenate/1
  Vector Concatenate/1 -> PARA_OUT/1
  Delay/1 -> Vector Concatenate/2, Delay1/1
  Constant/1 -> Delay1/2, Delay/2

== system gm_rec_i2s/REC_I2S_FIFO/SIPO_32BIT_R/Subsystem/SIPO_16BIT1/SIPO_8BIT/SIPO_4BIT1/2BIT_SIPO ==
  SERIAL_IN : Inport
  Constant : Constant  OutDataTypeStr=boolean  SampleTime=-1
  Delay : Delay  DelayLength=1  InitialCondition=0  ShowEnablePort=on
      settings: InputPortMap=u0,e6
  Delay1 : Delay  DelayLength=1  InitialCondition=0  ShowEnablePort=on
      settings: InputPortMap=u0,e6
  Vector Concatenate : Concatenate
  PARA_OUT : Outport  VectorParamsAs1DForOutWhenUnconnected=off
  SERIAL_OUT : Outport  Port=2  VectorParamsAs1DForOutWhenUnconnected=off
  wires:
  SERIAL_IN/1 -> Delay/1
  Delay1/1 -> SERIAL_OUT/1, Vector Concatenate/1
  Vector Concatenate/1 -> PARA_OUT/1
  Delay/1 -> Vector Concatenate/2, Delay1/1
  Constant/1 -> Delay1/2, Delay/2

== system gm_rec_i2s/REC_I2S_FIFO/SIPO_32BIT_R/Subsystem/SIPO_16BIT1/SIPO_8BIT/SIPO_4BIT1/2BIT_SIPO1 ==
  SERIAL_IN : Inport
  Constant : Constant  OutDataTypeStr=boolean  SampleTime=-1
  Delay : Delay  DelayLength=1  InitialCondition=0  ShowEnablePort=on
      settings: InputPortMap=u0,e6
  Delay1 : Delay  DelayLength=1  InitialCondition=0  ShowEnablePort=on
      settings: InputPortMap=u0,e6
  Vector Concatenate : Concatenate
  PARA_OUT : Outport  VectorParamsAs1DForOutWhenUnconnected=off
  SERIAL_OUT : Outport  Port=2  VectorParamsAs1DForOutWhenUnconnected=off
  wires:
  SERIAL_IN/1 -> Delay/1
  Delay1/1 -> SERIAL_OUT/1, Vector Concatenate/1
  Vector Concatenate/1 -> PARA_OUT/1
  Delay/1 -> Vector Concatenate/2, Delay1/1
  Constant/1 -> Delay1/2, Delay/2

== system gm_rec_i2s/REC_I2S_FIFO/SIPO_32BIT_R/Subsystem/SIPO_16BIT1/SIPO_8BIT1/SIPO_4BIT/2BIT_SIPO ==
  SERIAL_IN : Inport
  Constant : Constant  OutDataTypeStr=boolean  SampleTime=-1
  Delay : Delay  DelayLength=1  InitialCondition=0  ShowEnablePort=on
      settings: InputPortMap=u0,e6
  Delay1 : Delay  DelayLength=1  InitialCondition=0  ShowEnablePort=on
      settings: InputPortMap=u0,e6
  Vector Concatenate : Concatenate
  PARA_OUT : Outport  VectorParamsAs1DForOutWhenUnconnected=off
  SERIAL_OUT : Outport  Port=2  VectorParamsAs1DForOutWhenUnconnected=off
  wires:
  SERIAL_IN/1 -> Delay/1
  Delay1/1 -> SERIAL_OUT/1, Vector Concatenate/1
  Vector Concatenate/1 -> PARA_OUT/1
  Delay/1 -> Vector Concatenate/2, Delay1/1
  Constant/1 -> Delay1/2, Delay/2

== system gm_rec_i2s/REC_I2S_FIFO/SIPO_32BIT_R/Subsystem/SIPO_16BIT1/SIPO_8BIT1/SIPO_4BIT/2BIT_SIPO1 ==
  SERIAL_IN : Inport
  Constant : Constant  OutDataTypeStr=boolean  SampleTime=-1
  Delay : Delay  DelayLength=1  InitialCondition=0  ShowEnablePort=on
      settings: InputPortMap=u0,e6
  Delay1 : Delay  DelayLength=1  InitialCondition=0  ShowEnablePort=on
      settings: InputPortMap=u0,e6
  Vector Concatenate : Concatenate
  PARA_OUT : Outport  VectorParamsAs1DForOutWhenUnconnected=off
  SERIAL_OUT : Outport  Port=2  VectorParamsAs1DForOutWhenUnconnected=off
  wires:
  SERIAL_IN/1 -> Delay/1
  Delay1/1 -> SERIAL_OUT/1, Vector Concatenate/1
  Vector Concatenate/1 -> PARA_OUT/1
  Delay/1 -> Vector Concatenate/2, Delay1/1
  Constant/1 -> Delay1/2, Delay/2

== system gm_rec_i2s/REC_I2S_FIFO/SIPO_32BIT_R/Subsystem/SIPO_16BIT1/SIPO_8BIT1/SIPO_4BIT1/2BIT_SIPO ==
  SERIAL_IN : Inport
  Constant : Constant  OutDataTypeStr=boolean  SampleTime=-1
  Delay : Delay  DelayLength=1  InitialCondition=0  ShowEnablePort=on
      settings: InputPortMap=u0,e6
  Delay1 : Delay  DelayLength=1  InitialCondition=0  ShowEnablePort=on
      settings: InputPortMap=u0,e6
  Vector Concatenate : Concatenate
  PARA_OUT : Outport  VectorParamsAs1DForOutWhenUnconnected=off
  SERIAL_OUT : Outport  Port=2  VectorParamsAs1DForOutWhenUnconnected=off
  wires:
  SERIAL_IN/1 -> Delay/1
  Delay1/1 -> SERIAL_OUT/1, Vector Concatenate/1
  Vector Concatenate/1 -> PARA_OUT/1
  Delay/1 -> Vector Concatenate/2, Delay1/1
  Constant/1 -> Delay1/2, Delay/2

== system gm_rec_i2s/REC_I2S_FIFO/SIPO_32BIT_R/Subsystem/SIPO_16BIT1/SIPO_8BIT1/SIPO_4BIT1/2BIT_SIPO1 ==
  SERIAL_IN : Inport
  Constant : Constant  OutDataTypeStr=boolean  SampleTime=-1
  Delay : Delay  DelayLength=1  InitialCondition=0  ShowEnablePort=on
      settings: InputPortMap=u0,e6
  Delay1 : Delay  DelayLength=1  InitialCondition=0  ShowEnablePort=on
      settings: InputPortMap=u0,e6
  Vector Concatenate : Concatenate
  PARA_OUT : Outport  VectorParamsAs1DForOutWhenUnconnected=off
  SERIAL_OUT : Outport  Port=2  VectorParamsAs1DForOutWhenUnconnected=off
  wires:
  SERIAL_IN/1 -> Delay/1
  Delay1/1 -> SERIAL_OUT/1, Vector Concatenate/1
  Vector Concatenate/1 -> PARA_OUT/1
  Delay/1 -> Vector Concatenate/2, Delay1/1
  Constant/1 -> Delay1/2, Delay/2

== system gm_rec_i2s/REC_I2S_NOFIFO/SIPO_32BIT_R/Subsystem/SIPO_16BIT/SIPO_8BIT/SIPO_4BIT/2BIT_SIPO ==
  SERIAL_IN : Inport
  Constant : Constant  OutDataTypeStr=boolean  SampleTime=1
  Delay : Delay  DelayLength=1  InitialCondition=0  ShowEnablePort=on  SampleTime=1
      settings: InputPortMap=u0,e6
  Delay1 : Delay  DelayLength=1  InitialCondition=0  ShowEnablePort=on  SampleTime=1
      settings: InputPortMap=u0,e6
  Vector Concatenate : Concatenate
  PARA_OUT : Outport  VectorParamsAs1DForOutWhenUnconnected=off
  SERIAL_OUT : Outport  Port=2  VectorParamsAs1DForOutWhenUnconnected=off
  wires:
  SERIAL_IN/1 -> Delay/1
  Delay1/1 -> SERIAL_OUT/1, Vector Concatenate/1
  Vector Concatenate/1 -> PARA_OUT/1
  Delay/1 -> Vector Concatenate/2, Delay1/1
  Constant/1 -> Delay1/2, Delay/2

== system gm_rec_i2s/REC_I2S_NOFIFO/SIPO_32BIT_R/Subsystem/SIPO_16BIT/SIPO_8BIT/SIPO_4BIT/2BIT_SIPO1 ==
  SERIAL_IN : Inport
  Constant : Constant  OutDataTypeStr=boolean  SampleTime=1
  Delay : Delay  DelayLength=1  InitialCondition=0  ShowEnablePort=on  SampleTime=1
      settings: InputPortMap=u0,e6
  Delay1 : Delay  DelayLength=1  InitialCondition=0  ShowEnablePort=on  SampleTime=1
      settings: InputPortMap=u0,e6
  Vector Concatenate : Concatenate
  PARA_OUT : Outport  VectorParamsAs1DForOutWhenUnconnected=off
  SERIAL_OUT : Outport  Port=2  VectorParamsAs1DForOutWhenUnconnected=off
  wires:
  SERIAL_IN/1 -> Delay/1
  Delay1/1 -> SERIAL_OUT/1, Vector Concatenate/1
  Vector Concatenate/1 -> PARA_OUT/1
  Delay/1 -> Vector Concatenate/2, Delay1/1
  Constant/1 -> Delay1/2, Delay/2

== system gm_rec_i2s/REC_I2S_NOFIFO/SIPO_32BIT_R/Subsystem/SIPO_16BIT/SIPO_8BIT/SIPO_4BIT1/2BIT_SIPO ==
  SERIAL_IN : Inport
  Constant : Constant  OutDataTypeStr=boolean  SampleTime=1
  Delay : Delay  DelayLength=1  InitialCondition=0  ShowEnablePort=on  SampleTime=1
      settings: InputPortMap=u0,e6
  Delay1 : Delay  DelayLength=1  InitialCondition=0  ShowEnablePort=on  SampleTime=1
      settings: InputPortMap=u0,e6
  Vector Concatenate : Concatenate
  PARA_OUT : Outport  VectorParamsAs1DForOutWhenUnconnected=off
  SERIAL_OUT : Outport  Port=2  VectorParamsAs1DForOutWhenUnconnected=off
  wires:
  SERIAL_IN/1 -> Delay/1
  Delay1/1 -> SERIAL_OUT/1, Vector Concatenate/1
  Vector Concatenate/1 -> PARA_OUT/1
  Delay/1 -> Vector Concatenate/2, Delay1/1
  Constant/1 -> Delay1/2, Delay/2

== system gm_rec_i2s/REC_I2S_NOFIFO/SIPO_32BIT_R/Subsystem/SIPO_16BIT/SIPO_8BIT/SIPO_4BIT1/2BIT_SIPO1 ==
  SERIAL_IN : Inport
  Constant : Constant  OutDataTypeStr=boolean  SampleTime=1
  Delay : Delay  DelayLength=1  InitialCondition=0  ShowEnablePort=on  SampleTime=1
      settings: InputPortMap=u0,e6
  Delay1 : Delay  DelayLength=1  InitialCondition=0  ShowEnablePort=on  SampleTime=1
      settings: InputPortMap=u0,e6
  Vector Concatenate : Concatenate
  PARA_OUT : Outport  VectorParamsAs1DForOutWhenUnconnected=off
  SERIAL_OUT : Outport  Port=2  VectorParamsAs1DForOutWhenUnconnected=off
  wires:
  SERIAL_IN/1 -> Delay/1
  Delay1/1 -> SERIAL_OUT/1, Vector Concatenate/1
  Vector Concatenate/1 -> PARA_OUT/1
  Delay/1 -> Vector Concatenate/2, Delay1/1
  Constant/1 -> Delay1/2, Delay/2

== system gm_rec_i2s/REC_I2S_NOFIFO/SIPO_32BIT_R/Subsystem/SIPO_16BIT/SIPO_8BIT1/SIPO_4BIT/2BIT_SIPO ==
  SERIAL_IN : Inport
  Constant : Constant  OutDataTypeStr=boolean  SampleTime=1
  Delay : Delay  DelayLength=1  InitialCondition=0  ShowEnablePort=on  SampleTime=1
      settings: InputPortMap=u0,e6
  Delay1 : Delay  DelayLength=1  InitialCondition=0  ShowEnablePort=on  SampleTime=1
      settings: InputPortMap=u0,e6
  Vector Concatenate : Concatenate
  PARA_OUT : Outport  VectorParamsAs1DForOutWhenUnconnected=off
  SERIAL_OUT : Outport  Port=2  VectorParamsAs1DForOutWhenUnconnected=off
  wires:
  SERIAL_IN/1 -> Delay/1
  Delay1/1 -> SERIAL_OUT/1, Vector Concatenate/1
  Vector Concatenate/1 -> PARA_OUT/1
  Delay/1 -> Vector Concatenate/2, Delay1/1
  Constant/1 -> Delay1/2, Delay/2

== system gm_rec_i2s/REC_I2S_NOFIFO/SIPO_32BIT_R/Subsystem/SIPO_16BIT/SIPO_8BIT1/SIPO_4BIT/2BIT_SIPO1 ==
  SERIAL_IN : Inport
  Constant : Constant  OutDataTypeStr=boolean  SampleTime=1
  Delay : Delay  DelayLength=1  InitialCondition=0  ShowEnablePort=on  SampleTime=1
      settings: InputPortMap=u0,e6
  Delay1 : Delay  DelayLength=1  InitialCondition=0  ShowEnablePort=on  SampleTime=1
      settings: InputPortMap=u0,e6
  Vector Concatenate : Concatenate
  PARA_OUT : Outport  VectorParamsAs1DForOutWhenUnconnected=off
  SERIAL_OUT : Outport  Port=2  VectorParamsAs1DForOutWhenUnconnected=off
  wires:
  SERIAL_IN/1 -> Delay/1
  Delay1/1 -> SERIAL_OUT/1, Vector Concatenate/1
  Vector Concatenate/1 -> PARA_OUT/1
  Delay/1 -> Vector Concatenate/2, Delay1/1
  Constant/1 -> Delay1/2, Delay/2

== system gm_rec_i2s/REC_I2S_NOFIFO/SIPO_32BIT_R/Subsystem/SIPO_16BIT/SIPO_8BIT1/SIPO_4BIT1/2BIT_SIPO ==
  SERIAL_IN : Inport
  Constant : Constant  OutDataTypeStr=boolean  SampleTime=1
  Delay : Delay  DelayLength=1  InitialCondition=0  ShowEnablePort=on  SampleTime=1
      settings: InputPortMap=u0,e6
  Delay1 : Delay  DelayLength=1  InitialCondition=0  ShowEnablePort=on  SampleTime=1
      settings: InputPortMap=u0,e6
  Vector Concatenate : Concatenate
  PARA_OUT : Outport  VectorParamsAs1DForOutWhenUnconnected=off
  SERIAL_OUT : Outport  Port=2  VectorParamsAs1DForOutWhenUnconnected=off
  wires:
  SERIAL_IN/1 -> Delay/1
  Delay1/1 -> SERIAL_OUT/1, Vector Concatenate/1
  Vector Concatenate/1 -> PARA_OUT/1
  Delay/1 -> Vector Concatenate/2, Delay1/1
  Constant/1 -> Delay1/2, Delay/2

== system gm_rec_i2s/REC_I2S_NOFIFO/SIPO_32BIT_R/Subsystem/SIPO_16BIT/SIPO_8BIT1/SIPO_4BIT1/2BIT_SIPO1 ==
  SERIAL_IN : Inport
  Constant : Constant  OutDataTypeStr=boolean  SampleTime=1
  Delay : Delay  DelayLength=1  InitialCondition=0  ShowEnablePort=on  SampleTime=1
      settings: InputPortMap=u0,e6
  Delay1 : Delay  DelayLength=1  InitialCondition=0  ShowEnablePort=on  SampleTime=1
      settings: InputPortMap=u0,e6
  Vector Concatenate : Concatenate
  PARA_OUT : Outport  VectorParamsAs1DForOutWhenUnconnected=off
  SERIAL_OUT : Outport  Port=2  VectorParamsAs1DForOutWhenUnconnected=off
  wires:
  SERIAL_IN/1 -> Delay/1
  Delay1/1 -> SERIAL_OUT/1, Vector Concatenate/1
  Vector Concatenate/1 -> PARA_OUT/1
  Delay/1 -> Vector Concatenate/2, Delay1/1
  Constant/1 -> Delay1/2, Delay/2

== system gm_rec_i2s/REC_I2S_NOFIFO/SIPO_32BIT_R/Subsystem/SIPO_16BIT1/SIPO_8BIT/SIPO_4BIT/2BIT_SIPO ==
  SERIAL_IN : Inport
  Constant : Constant  OutDataTypeStr=boolean  SampleTime=1
  Delay : Delay  DelayLength=1  InitialCondition=0  ShowEnablePort=on  SampleTime=1
      settings: InputPortMap=u0,e6
  Delay1 : Delay  DelayLength=1  InitialCondition=0  ShowEnablePort=on  SampleTime=1
      settings: InputPortMap=u0,e6
  Vector Concatenate : Concatenate
  PARA_OUT : Outport  VectorParamsAs1DForOutWhenUnconnected=off
  SERIAL_OUT : Outport  Port=2  VectorParamsAs1DForOutWhenUnconnected=off
  wires:
  SERIAL_IN/1 -> Delay/1
  Delay1/1 -> SERIAL_OUT/1, Vector Concatenate/1
  Vector Concatenate/1 -> PARA_OUT/1
  Delay/1 -> Vector Concatenate/2, Delay1/1
  Constant/1 -> Delay1/2, Delay/2

== system gm_rec_i2s/REC_I2S_NOFIFO/SIPO_32BIT_R/Subsystem/SIPO_16BIT1/SIPO_8BIT/SIPO_4BIT/2BIT_SIPO1 ==
  SERIAL_IN : Inport
  Constant : Constant  OutDataTypeStr=boolean  SampleTime=1
  Delay : Delay  DelayLength=1  InitialCondition=0  ShowEnablePort=on  SampleTime=1
      settings: InputPortMap=u0,e6
  Delay1 : Delay  DelayLength=1  InitialCondition=0  ShowEnablePort=on  SampleTime=1
      settings: InputPortMap=u0,e6
  Vector Concatenate : Concatenate
  PARA_OUT : Outport  VectorParamsAs1DForOutWhenUnconnected=off
  SERIAL_OUT : Outport  Port=2  VectorParamsAs1DForOutWhenUnconnected=off
  wires:
  SERIAL_IN/1 -> Delay/1
  Delay1/1 -> SERIAL_OUT/1, Vector Concatenate/1
  Vector Concatenate/1 -> PARA_OUT/1
  Delay/1 -> Vector Concatenate/2, Delay1/1
  Constant/1 -> Delay1/2, Delay/2

== system gm_rec_i2s/REC_I2S_NOFIFO/SIPO_32BIT_R/Subsystem/SIPO_16BIT1/SIPO_8BIT/SIPO_4BIT1/2BIT_SIPO ==
  SERIAL_IN : Inport
  Constant : Constant  OutDataTypeStr=boolean  SampleTime=1
  Delay : Delay  DelayLength=1  InitialCondition=0  ShowEnablePort=on  SampleTime=1
      settings: InputPortMap=u0,e6
  Delay1 : Delay  DelayLength=1  InitialCondition=0  ShowEnablePort=on  SampleTime=1
      settings: InputPortMap=u0,e6
  Vector Concatenate : Concatenate
  PARA_OUT : Outport  VectorParamsAs1DForOutWhenUnconnected=off
  SERIAL_OUT : Outport  Port=2  VectorParamsAs1DForOutWhenUnconnected=off
  wires:
  SERIAL_IN/1 -> Delay/1
  Delay1/1 -> SERIAL_OUT/1, Vector Concatenate/1
  Vector Concatenate/1 -> PARA_OUT/1
  Delay/1 -> Vector Concatenate/2, Delay1/1
  Constant/1 -> Delay1/2, Delay/2

== system gm_rec_i2s/REC_I2S_NOFIFO/SIPO_32BIT_R/Subsystem/SIPO_16BIT1/SIPO_8BIT/SIPO_4BIT1/2BIT_SIPO1 ==
  SERIAL_IN : Inport
  Constant : Constant  OutDataTypeStr=boolean  SampleTime=1
  Delay : Delay  DelayLength=1  InitialCondition=0  ShowEnablePort=on  SampleTime=1
      settings: InputPortMap=u0,e6
  Delay1 : Delay  DelayLength=1  InitialCondition=0  ShowEnablePort=on  SampleTime=1
      settings: InputPortMap=u0,e6
  Vector Concatenate : Concatenate
  PARA_OUT : Outport  VectorParamsAs1DForOutWhenUnconnected=off
  SERIAL_OUT : Outport  Port=2  VectorParamsAs1DForOutWhenUnconnected=off
  wires:
  SERIAL_IN/1 -> Delay/1
  Delay1/1 -> SERIAL_OUT/1, Vector Concatenate/1
  Vector Concatenate/1 -> PARA_OUT/1
  Delay/1 -> Vector Concatenate/2, Delay1/1
  Constant/1 -> Delay1/2, Delay/2

== system gm_rec_i2s/REC_I2S_NOFIFO/SIPO_32BIT_R/Subsystem/SIPO_16BIT1/SIPO_8BIT1/SIPO_4BIT/2BIT_SIPO ==
  SERIAL_IN : Inport
  Constant : Constant  OutDataTypeStr=boolean  SampleTime=1
  Delay : Delay  DelayLength=1  InitialCondition=0  ShowEnablePort=on  SampleTime=1
      settings: InputPortMap=u0,e6
  Delay1 : Delay  DelayLength=1  InitialCondition=0  ShowEnablePort=on  SampleTime=1
      settings: InputPortMap=u0,e6
  Vector Concatenate : Concatenate
  PARA_OUT : Outport  VectorParamsAs1DForOutWhenUnconnected=off
  SERIAL_OUT : Outport  Port=2  VectorParamsAs1DForOutWhenUnconnected=off
  wires:
  SERIAL_IN/1 -> Delay/1
  Delay1/1 -> SERIAL_OUT/1, Vector Concatenate/1
  Vector Concatenate/1 -> PARA_OUT/1
  Delay/1 -> Vector Concatenate/2, Delay1/1
  Constant/1 -> Delay1/2, Delay/2

== system gm_rec_i2s/REC_I2S_NOFIFO/SIPO_32BIT_R/Subsystem/SIPO_16BIT1/SIPO_8BIT1/SIPO_4BIT/2BIT_SIPO1 ==
  SERIAL_IN : Inport
  Constant : Constant  OutDataTypeStr=boolean  SampleTime=1
  Delay : Delay  DelayLength=1  InitialCondition=0  ShowEnablePort=on  SampleTime=1
      settings: InputPortMap=u0,e6
  Delay1 : Delay  DelayLength=1  InitialCondition=0  ShowEnablePort=on  SampleTime=1
      settings: InputPortMap=u0,e6
  Vector Concatenate : Concatenate
  PARA_OUT : Outport  VectorParamsAs1DForOutWhenUnconnected=off
  SERIAL_OUT : Outport  Port=2  VectorParamsAs1DForOutWhenUnconnected=off
  wires:
  SERIAL_IN/1 -> Delay/1
  Delay1/1 -> SERIAL_OUT/1, Vector Concatenate/1
  Vector Concatenate/1 -> PARA_OUT/1
  Delay/1 -> Vector Concatenate/2, Delay1/1
  Constant/1 -> Delay1/2, Delay/2

== system gm_rec_i2s/REC_I2S_NOFIFO/SIPO_32BIT_R/Subsystem/SIPO_16BIT1/SIPO_8BIT1/SIPO_4BIT1/2BIT_SIPO ==
  SERIAL_IN : Inport
  Constant : Constant  OutDataTypeStr=boolean  SampleTime=1
  Delay : Delay  DelayLength=1  InitialCondition=0  ShowEnablePort=on  SampleTime=1
      settings: InputPortMap=u0,e6
  Delay1 : Delay  DelayLength=1  InitialCondition=0  ShowEnablePort=on  SampleTime=1
      settings: InputPortMap=u0,e6
  Vector Concatenate : Concatenate
  PARA_OUT : Outport  VectorParamsAs1DForOutWhenUnconnected=off
  SERIAL_OUT : Outport  Port=2  VectorParamsAs1DForOutWhenUnconnected=off
  wires:
  SERIAL_IN/1 -> Delay/1
  Delay1/1 -> SERIAL_OUT/1, Vector Concatenate/1
  Vector Concatenate/1 -> PARA_OUT/1
  Delay/1 -> Vector Concatenate/2, Delay1/1
  Constant/1 -> Delay1/2, Delay/2

== system gm_rec_i2s/REC_I2S_NOFIFO/SIPO_32BIT_R/Subsystem/SIPO_16BIT1/SIPO_8BIT1/SIPO_4BIT1/2BIT_SIPO1 ==
  SERIAL_IN : Inport
  Constant : Constant  OutDataTypeStr=boolean  SampleTime=1
  Delay : Delay  DelayLength=1  InitialCondition=0  ShowEnablePort=on  SampleTime=1
      settings: InputPortMap=u0,e6
  Delay1 : Delay  DelayLength=1  InitialCondition=0  ShowEnablePort=on  SampleTime=1
      settings: InputPortMap=u0,e6
  Vector Concatenate : Concatenate
  PARA_OUT : Outport  VectorParamsAs1DForOutWhenUnconnected=off
  SERIAL_OUT : Outport  Port=2  VectorParamsAs1DForOutWhenUnconnected=off
  wires:
  SERIAL_IN/1 -> Delay/1
  Delay1/1 -> SERIAL_OUT/1, Vector Concatenate/1
  Vector Concatenate/1 -> PARA_OUT/1
  Delay/1 -> Vector Concatenate/2, Delay1/1
  Constant/1 -> Delay1/2, Delay/2

== system gm_rec_i2s/REC_I2S_NOFIFO/SIPO_32BIT_R1/Subsystem/SIPO_16BIT/SIPO_8BIT/SIPO_4BIT/2BIT_SIPO ==
  SERIAL_IN : Inport
  Constant : Constant  OutDataTypeStr=boolean  SampleTime=1
  Delay : Delay  DelayLength=1  InitialCondition=0  ShowEnablePort=on  SampleTime=1
      settings: InputPortMap=u0,e6
  Delay1 : Delay  DelayLength=1  InitialCondition=0  ShowEnablePort=on  SampleTime=1
      settings: InputPortMap=u0,e6
  Vector Concatenate : Concatenate
  PARA_OUT : Outport  VectorParamsAs1DForOutWhenUnconnected=off
  SERIAL_OUT : Outport  Port=2  VectorParamsAs1DForOutWhenUnconnected=off
  wires:
  SERIAL_IN/1 -> Delay/1
  Delay1/1 -> SERIAL_OUT/1, Vector Concatenate/1
  Vector Concatenate/1 -> PARA_OUT/1
  Delay/1 -> Vector Concatenate/2, Delay1/1
  Constant/1 -> Delay1/2, Delay/2
